simulink model "BLDC_FOC_Model"  (R2022b)
settings: Solver=FixedStepDiscrete  StartTime=0.0  StopTime=0.5  FixedStep=1e-06  RelTol=1e-3
settings Model: Creator=16664  LastModifiedBy=16664
settings DataIOCC: SaveFormat=StructureWithTime

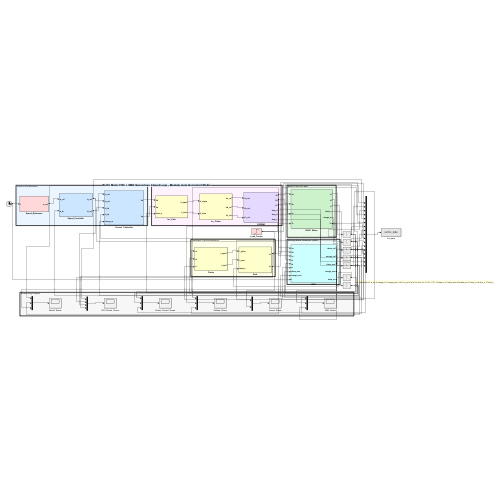
[thumbnail: Simulink's stored preview of the top-level diagram]
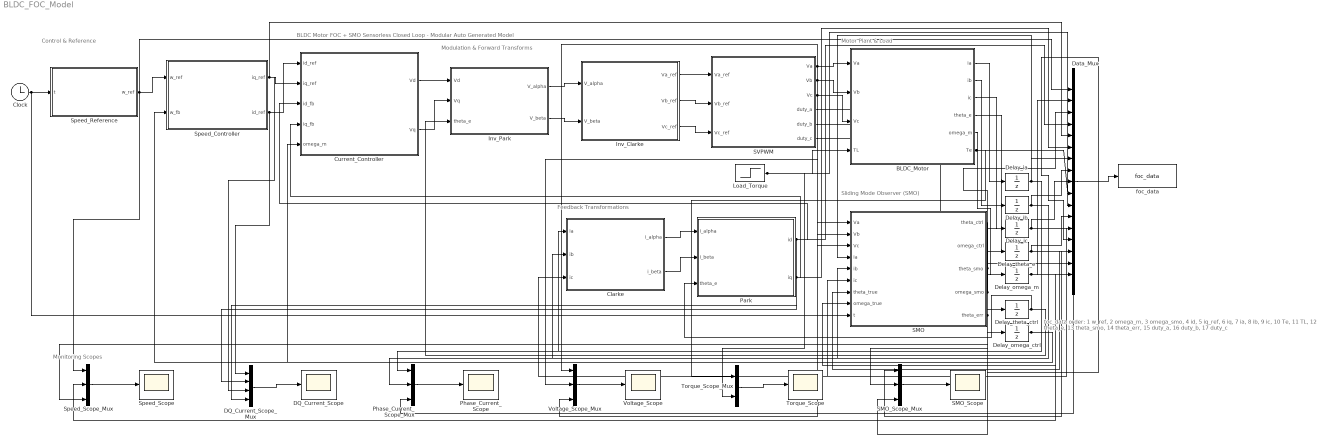
== system BLDC_FOC_Model ==
  note: BLDC Motor FOC + SMO Sensorless Closed Loop - Modular Auto Generated Model
  note: foc_data order:\n1 w_ref, 2 omega_m, 3 omega_smo, 4 id, 5 iq_ref, 6 iq,\n7 ia, 8 ib, 9 ic, 10 Te, 11 TL, 12 theta_e, 13 theta_smo,\n14 theta_err, 15 duty_a, 16 duty_b, 17 duty_c
  note: Control & Reference
  note: Modulation & Forward Transforms
  note: Motor Plant & Load
  note: Feedback Transformations
  note: Sliding Mode Observer (SMO)
  note: Monitoring Scopes
  BLDC_Motor : Subsystem
  Clarke : Subsystem
  Clock : Clock
  Current_Controller : Subsystem
  DQ_Current_Scope : Scope
  DQ_Current_Scope_Mux : Mux
  Data_Mux : Mux  Inputs=17
  Delay_ia : UnitDelay  SampleTime=1e-06  HasFrameUpgradeWarning=on
  Delay_ib : UnitDelay  SampleTime=1e-06  HasFrameUpgradeWarning=on
  Delay_ic : UnitDelay  SampleTime=1e-06  HasFrameUpgradeWarning=on
  Delay_omega_ctrl : UnitDelay  SampleTime=1e-06  HasFrameUpgradeWarning=on
  Delay_omega_m : UnitDelay  SampleTime=1e-06  HasFrameUpgradeWarning=on
  Delay_theta_ctrl : UnitDelay  SampleTime=1e-06  HasFrameUpgradeWarning=on
  Delay_theta_e : UnitDelay  SampleTime=1e-06  HasFrameUpgradeWarning=on
  Inv_Clarke : Subsystem
  Inv_Park : Subsystem
  Load_Torque : Step  Time=0.3  After=0.1  SampleTime=0
  Park : Subsystem
  Phase_Current_Scope : Scope
  Phase_Current_Scope_Mux : Mux  Inputs=3
  SMO : Subsystem
  SMO_Scope : Scope
  SMO_Scope_Mux : Mux  Inputs=3
  SVPWM : Subsystem
  Speed_Controller : Subsystem
  Speed_Reference : Subsystem
  Speed_Scope : Scope
  Speed_Scope_Mux : Mux  Inputs=3
  Torque_Scope : Scope
  Torque_Scope_Mux : Mux  Inputs=2
  Voltage_Scope : Scope
  Voltage_Scope_Mux : Mux  Inputs=3
  foc_data : ToWorkspace  VariableName=foc_data  SaveFormat=Structure With Time  SampleTime=-1
  wires:
  Clock/1 -> Speed_Reference/1(t), SMO/9(t)
  Speed_Reference/1(w_ref) -> Speed_Controller/1(w_ref), Speed_Scope_Mux/1, Data_Mux/1
  Delay_omega_ctrl/1 -> Speed_Controller/2(w_fb), Current_Controller/5(omega_m)
  Speed_Controller/2(id_ref) -> Current_Controller/1(id_ref), DQ_Current_Scope_Mux/1
  Speed_Controller/1(iq_ref) -> Current_Controller/2(iq_ref), DQ_Current_Scope_Mux/3, Data_Mux/5
  Park/1(id) -> Current_Controller/3(id_fb), DQ_Current_Scope_Mux/2, Data_Mux/4
  Park/2(iq) -> Current_Controller/4(iq_fb), DQ_Current_Scope_Mux/4, Data_Mux/6
  Current_Controller/1(Vd) -> Inv_Park/1(Vd)
  Current_Controller/2(Vq) -> Inv_Park/2(Vq)
  Delay_theta_ctrl/1 -> Inv_Park/3(theta_e), Park/3(theta_e)
  Inv_Park/1(V_alpha) -> Inv_Clarke/1(V_alpha)
  Inv_Park/2(V_beta) -> Inv_Clarke/2(V_beta)
  Inv_Clarke/1(Va_ref) -> SVPWM/1(Va_ref)
  Inv_Clarke/2(Vb_ref) -> SVPWM/2(Vb_ref)
  Inv_Clarke/3(Vc_ref) -> SVPWM/3(Vc_ref)
  SVPWM/1(Va) -> BLDC_Motor/1(Va), SMO/1(Va), Voltage_Scope_Mux/1
  SVPWM/2(Vb) -> BLDC_Motor/2(Vb), SMO/2(Vb), Voltage_Scope_Mux/2
  SVPWM/3(Vc) -> BLDC_Motor/3(Vc), SMO/3(Vc), Voltage_Scope_Mux/3
  Load_Torque/1 -> BLDC_Motor/4(TL), Torque_Scope_Mux/2, Data_Mux/11
  BLDC_Motor/1(ia) -> Delay_ia/1
  BLDC_Motor/2(ib) -> Delay_ib/1
  BLDC_Motor/3(ic) -> Delay_ic/1
  BLDC_Motor/4(theta_e) -> Delay_theta_e/1
  BLDC_Motor/5(omega_m) -> Delay_omega_m/1
  Delay_ia/1 -> Clarke/1(ia), SMO/4(ia), Phase_Current_Scope_Mux/1, Data_Mux/7
  Delay_ib/1 -> Clarke/2(ib), SMO/5(ib), Phase_Current_Scope_Mux/2, Data_Mux/8
  Delay_ic/1 -> Clarke/3(ic), SMO/6(ic), Phase_Current_Scope_Mux/3, Data_Mux/9
  Clarke/1(i_alpha) -> Park/1(i_alpha)
  Clarke/2(i_beta) -> Park/2(i_beta)
  Delay_theta_e/1 -> SMO/7(theta_true), SMO_Scope_Mux/1, Data_Mux/12
  Delay_omega_m/1 -> SMO/8(omega_true), Speed_Scope_Mux/2, Data_Mux/2
  SMO/1(theta_ctrl) -> Delay_theta_ctrl/1
  SMO/2(omega_ctrl) -> Delay_omega_ctrl/1
  SMO/4(omega_smo) -> Speed_Scope_Mux/3, Data_Mux/3
  Speed_Scope_Mux/1 -> Speed_Scope/1
  DQ_Current_Scope_Mux/1 -> DQ_Current_Scope/1
  Phase_Current_Scope_Mux/1 -> Phase_Current_Scope/1
  Voltage_Scope_Mux/1 -> Voltage_Scope/1
  BLDC_Motor/6(Te) -> Torque_Scope_Mux/1, Data_Mux/10
  Torque_Scope_Mux/1 -> Torque_Scope/1
  SMO/3(theta_smo) -> SMO_Scope_Mux/2, Data_Mux/13
  SMO/5(theta_err) -> SMO_Scope_Mux/3, Data_Mux/14
  SMO_Scope_Mux/1 -> SMO_Scope/1
  SVPWM/4(duty_a) -> Data_Mux/15
  SVPWM/5(duty_b) -> Data_Mux/16
  SVPWM/6(duty_c) -> Data_Mux/17
  Data_Mux/1 -> foc_data/1

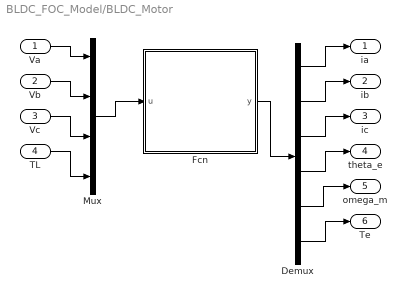
== system BLDC_FOC_Model/BLDC_Motor ==
  Va : Inport
  Vb : Inport  Port=2
  Vc : Inport  Port=3
  TL : Inport  Port=4
  Demux : Demux  Outputs=6
  Fcn : MATLAB Function  TreatAsAtomicUnit=on
  Mux : Mux
  ia : Outport
  ib : Outport  Port=2
  ic : Outport  Port=3
  theta_e : Outport  Port=4
  omega_m : Outport  Port=5
  Te : Outport  Port=6
  wires:
  Va/1 -> Mux/1
  Vb/1 -> Mux/2
  Vc/1 -> Mux/3
  TL/1 -> Mux/4
  Mux/1 -> Fcn/1(u)
  Fcn/1(y) -> Demux/1
  Demux/1 -> ia/1
  Demux/2 -> ib/1
  Demux/3 -> ic/1
  Demux/4 -> theta_e/1
  Demux/5 -> omega_m/1
  Demux/6 -> Te/1

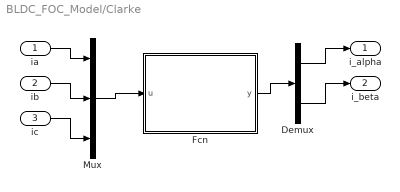
== system BLDC_FOC_Model/Clarke ==
  ia : Inport
  ib : Inport  Port=2
  ic : Inport  Port=3
  Demux : Demux  Outputs=2
  Fcn : MATLAB Function  TreatAsAtomicUnit=on
  Mux : Mux  Inputs=3
  i_alpha : Outport
  i_beta : Outport  Port=2
  wires:
  ia/1 -> Mux/1
  ib/1 -> Mux/2
  ic/1 -> Mux/3
  Mux/1 -> Fcn/1(u)
  Fcn/1(y) -> Demux/1
  Demux/1 -> i_alpha/1
  Demux/2 -> i_beta/1

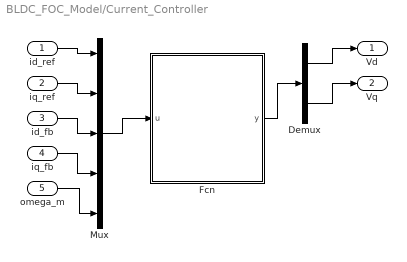
== system BLDC_FOC_Model/Current_Controller ==
  id_ref : Inport
  iq_ref : Inport  Port=2
  id_fb : Inport  Port=3
  iq_fb : Inport  Port=4
  omega_m : Inport  Port=5
  Demux : Demux  Outputs=2
  Fcn : MATLAB Function  TreatAsAtomicUnit=on
  Mux : Mux  Inputs=5
  Vd : Outport
  Vq : Outport  Port=2
  wires:
  id_ref/1 -> Mux/1
  iq_ref/1 -> Mux/2
  id_fb/1 -> Mux/3
  iq_fb/1 -> Mux/4
  omega_m/1 -> Mux/5
  Mux/1 -> Fcn/1(u)
  Fcn/1(y) -> Demux/1
  Demux/1 -> Vd/1
  Demux/2 -> Vq/1

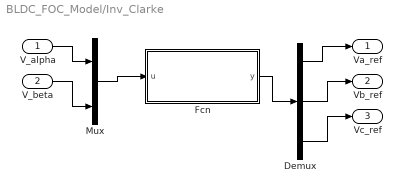
== system BLDC_FOC_Model/Inv_Clarke ==
  V_alpha : Inport
  V_beta : Inport  Port=2
  Demux : Demux  Outputs=3
  Fcn : MATLAB Function  TreatAsAtomicUnit=on
  Mux : Mux  Inputs=2
  Va_ref : Outport
  Vb_ref : Outport  Port=2
  Vc_ref : Outport  Port=3
  wires:
  V_alpha/1 -> Mux/1
  V_beta/1 -> Mux/2
  Mux/1 -> Fcn/1(u)
  Fcn/1(y) -> Demux/1
  Demux/1 -> Va_ref/1
  Demux/2 -> Vb_ref/1
  Demux/3 -> Vc_ref/1

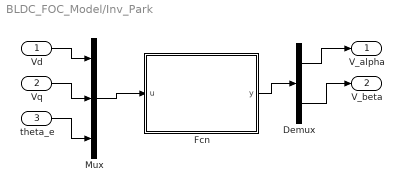
== system BLDC_FOC_Model/Inv_Park ==
  Vd : Inport
  Vq : Inport  Port=2
  theta_e : Inport  Port=3
  Demux : Demux  Outputs=2
  Fcn : MATLAB Function  TreatAsAtomicUnit=on
  Mux : Mux  Inputs=3
  V_alpha : Outport
  V_beta : Outport  Port=2
  wires:
  Vd/1 -> Mux/1
  Vq/1 -> Mux/2
  theta_e/1 -> Mux/3
  Mux/1 -> Fcn/1(u)
  Fcn/1(y) -> Demux/1
  Demux/1 -> V_alpha/1
  Demux/2 -> V_beta/1

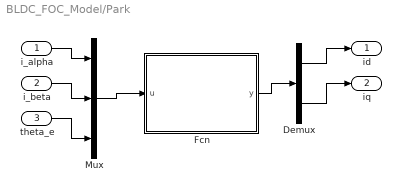
== system BLDC_FOC_Model/Park ==
  i_alpha : Inport
  i_beta : Inport  Port=2
  theta_e : Inport  Port=3
  Demux : Demux  Outputs=2
  Fcn : MATLAB Function  TreatAsAtomicUnit=on
  Mux : Mux  Inputs=3
  id : Outport
  iq : Outport  Port=2
  wires:
  i_alpha/1 -> Mux/1
  i_beta/1 -> Mux/2
  theta_e/1 -> Mux/3
  Mux/1 -> Fcn/1(u)
  Fcn/1(y) -> Demux/1
  Demux/1 -> id/1
  Demux/2 -> iq/1

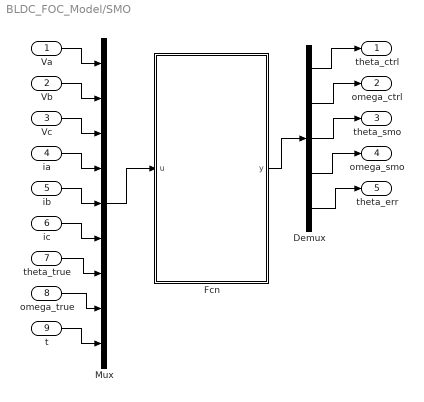
== system BLDC_FOC_Model/SMO ==
  Va : Inport
  Vb : Inport  Port=2
  Vc : Inport  Port=3
  ia : Inport  Port=4
  ib : Inport  Port=5
  ic : Inport  Port=6
  theta_true : Inport  Port=7
  omega_true : Inport  Port=8
  t : Inport  Port=9
  Demux : Demux  Outputs=5
  Fcn : MATLAB Function  TreatAsAtomicUnit=on
  Mux : Mux  Inputs=9
  theta_ctrl : Outport
  omega_ctrl : Outport  Port=2
  theta_smo : Outport  Port=3
  omega_smo : Outport  Port=4
  theta_err : Outport  Port=5
  wires:
  Va/1 -> Mux/1
  Vb/1 -> Mux/2
  Vc/1 -> Mux/3
  ia/1 -> Mux/4
  ib/1 -> Mux/5
  ic/1 -> Mux/6
  theta_true/1 -> Mux/7
  omega_true/1 -> Mux/8
  t/1 -> Mux/9
  Mux/1 -> Fcn/1(u)
  Fcn/1(y) -> Demux/1
  Demux/1 -> theta_ctrl/1
  Demux/2 -> omega_ctrl/1
  Demux/3 -> theta_smo/1
  Demux/4 -> omega_smo/1
  Demux/5 -> theta_err/1

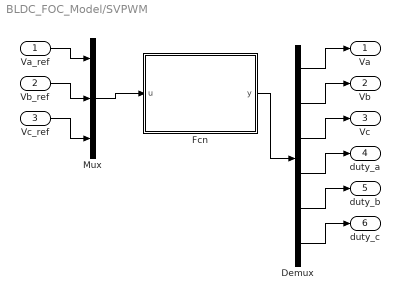
== system BLDC_FOC_Model/SVPWM ==
  Va_ref : Inport
  Vb_ref : Inport  Port=2
  Vc_ref : Inport  Port=3
  Demux : Demux  Outputs=6
  Fcn : MATLAB Function  TreatAsAtomicUnit=on
  Mux : Mux  Inputs=3
  Va : Outport
  Vb : Outport  Port=2
  Vc : Outport  Port=3
  duty_a : Outport  Port=4
  duty_b : Outport  Port=5
  duty_c : Outport  Port=6
  wires:
  Va_ref/1 -> Mux/1
  Vb_ref/1 -> Mux/2
  Vc_ref/1 -> Mux/3
  Mux/1 -> Fcn/1(u)
  Fcn/1(y) -> Demux/1
  Demux/1 -> Va/1
  Demux/2 -> Vb/1
  Demux/3 -> Vc/1
  Demux/4 -> duty_a/1
  Demux/5 -> duty_b/1
  Demux/6 -> duty_c/1

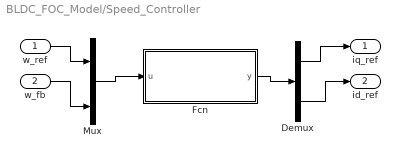
== system BLDC_FOC_Model/Speed_Controller ==
  w_ref : Inport
  w_fb : Inport  Port=2
  Demux : Demux  Outputs=2
  Fcn : MATLAB Function  TreatAsAtomicUnit=on
  Mux : Mux  Inputs=2
  iq_ref : Outport
  id_ref : Outport  Port=2
  wires:
  w_ref/1 -> Mux/1
  w_fb/1 -> Mux/2
  Mux/1 -> Fcn/1(u)
  Fcn/1(y) -> Demux/1
  Demux/1 -> iq_ref/1
  Demux/2 -> id_ref/1

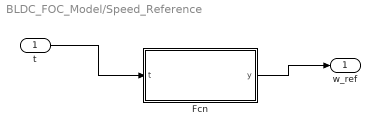
== system BLDC_FOC_Model/Speed_Reference ==
  t : Inport
  Fcn : MATLAB Function  TreatAsAtomicUnit=on
  w_ref : Outport
  wires:
  t/1 -> Fcn/1(t)
  Fcn/1(y) -> w_ref/1

== matlab function BLDC_FOC_Model/Speed_Reference/Fcn ==
  data: t input; y output
function y = fcn(t)
%#codegen
if t < 0.01
    y = 0;
elseif t < 0.06
    y = 2094.395102393195 * (t - 0.01);
else
    y = 104.71975511965977;
end
end

== matlab function BLDC_FOC_Model/Current_Controller/Fcn ==
  data: u input; y output
function y = fcn(u)
%#codegen
persistent int_id int_iq counter vd vq
if isempty(int_id), int_id=0; int_iq=0; counter=0; vd=0; vq=0; end
dt=9.9999999999999995e-07; Ts=5.0000000000000002e-05; Vdc=24; Ld=0.00080000000000000004; Lq=0.00080000000000000004; flux=0.017500000000000002; pp=4;
id_ref=u(1); iq_ref=u(2); id=u(3); iq=u(4); omega_m=u(5); counter=counter+dt;
if counter >= Ts
    counter=0;
    err=id_ref-id; int_id=int_id+1000*err*Ts; unsat=5*err+int_id; vd=min(12,max(-12,unsat)); if vd~=unsat, int_id=int_id-1000*err*Ts; end
    err=iq_ref-iq; int_iq=int_iq+1000*err*Ts; unsat=5*err+int_iq; vq=min(12,max(-12,unsat)); if vq~=unsat, int_iq=int_iq-1000*err*Ts; end
    omega_e=omega_m*pp; vd=vd-omega_e*Lq*iq; vq=vq+omega_e*Ld*id+omega_e*flux;
    Vmax=Vdc/sqrt(3); Vmag=sqrt(vd*vd+vq*vq); if Vmag>Vmax, vd=vd*Vmax/Vmag; vq=vq*Vmax/Vmag; end
end
y=zeros(2,1); y(1)=vd; y(2)=vq;
end

== matlab function BLDC_FOC_Model/Inv_Park/Fcn ==
  data: u input; y output
function y = fcn(u)
%#codegen
vd=u(1); vq=u(2); th=u(3);
y=zeros(2,1); y(1)=vd*cos(th)-vq*sin(th); y(2)=vd*sin(th)+vq*cos(th);
end

== matlab function BLDC_FOC_Model/Inv_Clarke/Fcn ==
  data: u input; y output
function y = fcn(u)
%#codegen
va=u(1); vb=u(2);
y=zeros(3,1); y(1)=va; y(2)=-0.5*va+sqrt(3)/2*vb; y(3)=-0.5*va-sqrt(3)/2*vb;
end

== matlab function BLDC_FOC_Model/SVPWM/Fcn ==
  data: u input; y output
function y = fcn(u)
%#codegen
Vdc=24; va=u(1); vb=u(2); vc=u(3);
vmax=max(max(va,vb),vc); vmin=min(min(va,vb),vc); voff=-0.5*(vmax+vmin);
da=min(1,max(0,0.5+(va+voff)/Vdc)); db=min(1,max(0,0.5+(vb+voff)/Vdc)); dc=min(1,max(0,0.5+(vc+voff)/Vdc));
y=zeros(6,1); y(1)=(2*da-1)*Vdc/2; y(2)=(2*db-1)*Vdc/2; y(3)=(2*dc-1)*Vdc/2; y(4)=da; y(5)=db; y(6)=dc;
end

== matlab function BLDC_FOC_Model/BLDC_Motor/Fcn ==
  data: u input; y output
function y = fcn(u)
%#codegen
persistent ia ib ic th wm
if isempty(ia), ia=0; ib=0; ic=0; th=0; wm=0; end
dt=9.9999999999999995e-07; Rs=0.5; Ld=0.00080000000000000004; Lq=0.00080000000000000004; flux=0.017500000000000002; pp=4; J=0.0001; B=0.0001;
va=u(1); vb=u(2); vc=u(3); TL=u(4); we=wm*pp;
valpha=(2/3)*(va-0.5*vb-0.5*vc); vbeta=(2/3)*(sqrt(3)/2*vb-sqrt(3)/2*vc);
vd=valpha*cos(th)+vbeta*sin(th); vq=-valpha*sin(th)+vbeta*cos(th);
ialpha=(2/3)*(ia-0.5*ib-0.5*ic); ibeta=(2/3)*(sqrt(3)/2*ib-sqrt(3)/2*ic);
id=ialpha*cos(th)+ibeta*sin(th); iq=-ialpha*sin(th)+ibeta*cos(th);
did=(vd-Rs*id+we*Lq*iq)/Ld; diq=(vq-Rs*iq-we*Ld*id-we*flux)/Lq;
idn=id+did*dt; iqn=iq+diq*dt; Te=1.5*pp*(flux*iqn+(Ld-Lq)*idn*iqn);
wm=wm+(Te-TL-B*wm)/J*dt; th=mod(th+wm*pp*dt,2*pi);
ialpha=idn*cos(th)-iqn*sin(th); ibeta=idn*sin(th)+iqn*cos(th);
ia=ialpha; ib=-0.5*ialpha+sqrt(3)/2*ibeta; ic=-0.5*ialpha-sqrt(3)/2*ibeta;
y=zeros(6,1); y(1)=ia; y(2)=ib; y(3)=ic; y(4)=th; y(5)=wm; y(6)=Te;
end

== matlab function BLDC_FOC_Model/Clarke/Fcn ==
  data: u input; y output
function y = fcn(u)
%#codegen
ia=u(1); ib=u(2); ic=u(3);
y=zeros(2,1); y(1)=(2/3)*(ia-0.5*ib-0.5*ic); y(2)=(2/3)*(sqrt(3)/2*ib-sqrt(3)/2*ic);
end

== matlab function BLDC_FOC_Model/Park/Fcn ==
  data: u input; y output
function y = fcn(u)
%#codegen
ialpha=u(1); ibeta=u(2); th=u(3);
y=zeros(2,1); y(1)=ialpha*cos(th)+ibeta*sin(th); y(2)=-ialpha*sin(th)+ibeta*cos(th);
end

== matlab function BLDC_FOC_Model/Speed_Controller/Fcn ==
  data: u input; y output
function y = fcn(u)
%#codegen
persistent integ counter iq_ref
if isempty(integ), integ=0; counter=0; iq_ref=0; end
dt=9.9999999999999995e-07; Ts=0.00050000000000000001; Kp=0.5; Ki=10; outMax=15; outMin=-15;
w_ref=u(1); w_fb=u(2); counter=counter+dt;
if counter >= Ts
    counter=0; err=w_ref-w_fb; integ=integ+Ki*err*Ts; unsat=Kp*err+integ;
    iq_ref=min(outMax,max(outMin,unsat));
    if iq_ref ~= unsat, integ=integ-Ki*err*Ts; end
end
y=zeros(2,1); y(1)=iq_ref; y(2)=0;
end

== matlab function BLDC_FOC_Model/SMO/Fcn ==
  data: u input; y output
function y = fcn(u)
%#codegen
persistent ih_a ih_b eh_a eh_b th_h we_h
if isempty(ih_a), ih_a=0; ih_b=0; eh_a=0; eh_b=0; th_h=0; we_h=0; end
Vdc=24; dt=9.9999999999999995e-07; Rs=0.5; Ls=0.00080000000000000004; pp=4; K=30; boundary=0.20000000000000001; emfCut=2000; speedCut=500; minEmf=0.050000000000000003; enableT=0.02; useSmo=1;
va=u(1); vb=u(2); vc=u(3); ia=u(4); ib=u(5); ic=u(6); th_true=u(7); wm_true=u(8); t=u(9);
v_alpha=(2/3)*(va-0.5*vb-0.5*vc); v_beta=(2/3)*(sqrt(3)/2*vb-sqrt(3)/2*vc);
i_alpha=(2/3)*(ia-0.5*ib-0.5*ic); i_beta=(2/3)*(sqrt(3)/2*ib-sqrt(3)/2*ic);
za=K*min(1,max(-1,(ih_a-i_alpha)/boundary)); zb=K*min(1,max(-1,(ih_b-i_beta)/boundary));
ih_a=ih_a+dt/Ls*(v_alpha-Rs*ih_a-za); ih_b=ih_b+dt/Ls*(v_beta-Rs*ih_b-zb);
a=dt*emfCut/(1+dt*emfCut); eh_a=eh_a+a*(za-eh_a); eh_b=eh_b+a*(zb-eh_b);
if sqrt(eh_a*eh_a+eh_b*eh_b) >= minEmf
    th_lpf=atan2(-eh_a,eh_b); th_raw=mod(th_lpf+atan2(we_h,emfCut),2*pi);
    dth=atan2(sin(th_raw-th_h),cos(th_raw-th_h)); omega_raw=dth/dt;
    b=dt*speedCut/(1+dt*speedCut); we_h=we_h+b*(omega_raw-we_h); th_h=th_raw;
end
if useSmo && t >= enableT, th_ctrl=th_h; wm_ctrl=we_h/pp; else, th_ctrl=th_true; wm_ctrl=wm_true; end
err=atan2(sin(th_h-th_true),cos(th_h-th_true));
y=zeros(5,1); y(1)=th_ctrl; y(2)=wm_ctrl; y(3)=th_h; y(4)=we_h/pp; y(5)=err;
end
